simulink model "beta_estimator_acceleration"  (R2022a)
settings: Solver=VariableStepAuto  StartTime=0.0  StopTime=10.0  FixedStep=1e-3  RelTol=1e-6  AbsTol=1e-10
values from neighbouring files (symbols this model uses):
  Den_PDa = [1,(Ts/Ta-2)/(Ts/Ta+2)]    [test_beta_estimator_acceleration.m]    (also in test_beta_estimator_compare.m)
  Num_PDa = [(Kpa*(2+Ts/Ta)+2*Kda/Ta)/(2+Ts/Ta),(-2*Kpa+Ts*Kpa/Ta-2*Kda/Ta)/(2+Ts/Ta)]    [test_beta_estimator_acceleration.m]    (also in test_beta_estimator_compare.m)
  Ts = 0.001    [test_beta_estimator_acceleration.m]    (also in test_beta_estimator_compare.m; test_beta_estimator_velocity.m)
  x0_acc = [0,0,0,0.1]    [test_beta_estimator_acceleration.m]    (also in test_beta_estimator_compare.m)
undefined symbols (not defined in the file or in its folder): DiscIntNeverNeededParam
settings Model: Creator=bascetta  LastModifiedBy=bascetta
settings SolverCC: AlgebraicLoopSolver=TrustRegion
settings DataIOCC: SaveOutput=off  SignalLogging=off  DSMLogging=off  SaveTime=off  ReturnWorkspaceOutputs=off
settings OptimizationCC: DefaultParameterBehavior=Inlined  PassReuseOutputArgsAs=Individual arguments  MaxStackSize=64  EfficientTunableParamExpr=on
settings DebuggingCC: ParameterTunabilityLossMsg=error  UnconnectedInputMsg=warning  UnconnectedOutputMsg=warning  UnconnectedLineMsg=warning  SFMachineParentedDataDiag=warning  ArithmeticOperatorsInVariantConditions=warning
settings HardwareCC: ProdBitPerPointer=32  ProdBitPerSizeT=32  ProdBitPerPtrDiffT=32  ProdLargestAtomicFloat=None  ProdIntDivRoundTo=Undefined  ProdEndianess=Unspecified  ProdWordSize=32  ProdHWDeviceType=Generic->Unspecified (assume 32-bit Generic)
settings SFSimCC: SimUseLocalCustomCode=off  MATLABDynamicMemAlloc=off  CustomCodeUndefinedFunction=UseInterfaceOnly
settings RTWCC: SystemTargetFile=ert.tlc  TemplateMakefile=ert_default_tmf  GenerateReport=on  RTWUseLocalCustomCode=off  Toolchain=Catkin  IncludeHyperlinkInReport=on  LaunchReport=on  GenerateTraceInfo=on  GenerateTraceReport=on  GenerateTraceReportSl=on  GenerateTraceReportSf=on  GenerateTraceReportEml=on  DLArmComputeVersion=19.05
settings CodeAppCC: ForceParamTrailComments=on  IgnoreCustomStorageClasses=off  OperatorAnnotations=on  SimulinkDataObjDesc=on  SFDataObjDesc=on  MATLABFcnDesc=on  InsertBlockDesc=on  StateflowObjectComments=on  MATLABSourceComments=on
settings ERTTargetCC: ERTCustomFileTemplate=example_file_process.tlc

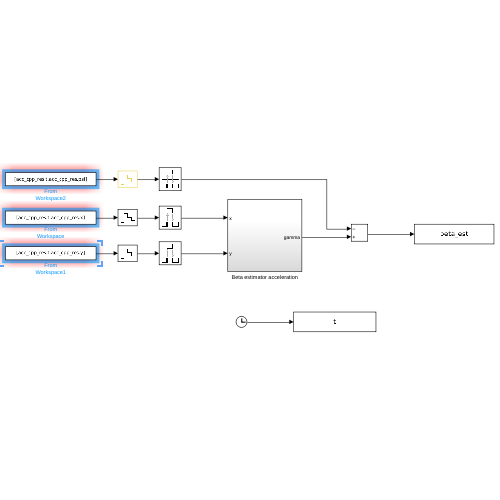
[thumbnail: Simulink's stored preview of the top-level diagram]
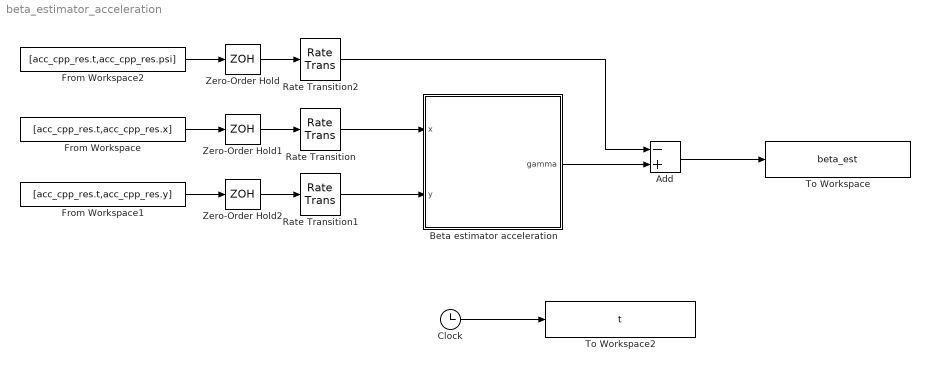
== system beta_estimator_acceleration ==
  Add : Sum  Inputs=-+
  Beta estimator acceleration : Subsystem  SystemSampleTime=Ts
  Clock : Clock
  From Workspace : FromWorkspace  VariableName=[acc_cpp_res.t,acc_cpp_res.x]  OutputAfterFinalValue=Holding final value
  From Workspace1 : FromWorkspace  VariableName=[acc_cpp_res.t,acc_cpp_res.y]  OutputAfterFinalValue=Holding final value
  From Workspace2 : FromWorkspace  VariableName=[acc_cpp_res.t,acc_cpp_res.psi]  OutputAfterFinalValue=Holding final value
  Rate Transition : RateTransition  OutPortSampleTime=Ts
  Rate Transition1 : RateTransition  OutPortSampleTime=Ts
  Rate Transition2 : RateTransition  OutPortSampleTime=Ts
  To Workspace : ToWorkspace  VariableName=beta_est  SampleTime=Ts
      settings: Save2DSignal=2-D array (concatenate along first dimension)
  To Workspace2 : ToWorkspace  VariableName=t  SampleTime=0.001
      settings: Save2DSignal=2-D array (concatenate along first dimension)
  Zero-Order Hold : ZeroOrderHold  SampleTime=0.01
  Zero-Order Hold1 : ZeroOrderHold  SampleTime=0.01
  Zero-Order Hold2 : ZeroOrderHold  SampleTime=0.01
  wires:
  Rate Transition/1 -> Beta estimator acceleration/1(x)
  Rate Transition1/1 -> Beta estimator acceleration/2(y)
  Beta estimator acceleration/1(gamma) -> Add/2
  Add/1 -> To Workspace/1
  Rate Transition2/1 -> Add/1
  Clock/1 -> To Workspace2/1
  From Workspace2/1 -> Zero-Order Hold/1
  Zero-Order Hold/1 -> Rate Transition2/1
  From Workspace/1 -> Zero-Order Hold1/1
  Zero-Order Hold1/1 -> Rate Transition/1
  From Workspace1/1 -> Zero-Order Hold2/1
  Zero-Order Hold2/1 -> Rate Transition1/1

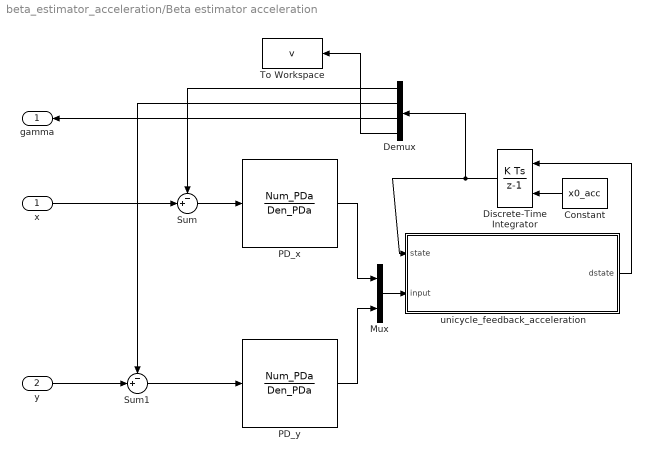
== system beta_estimator_acceleration/Beta estimator acceleration ==
  x : Inport
  y : Inport  Port=2
  Constant : Constant  Value=x0_acc
  Demux : Demux
  Discrete-Time Integrator : DiscreteIntegrator  InitialConditionSource=external  InitialCondition=[0 0 0 0.1]  SampleTime=Ts  ICPrevOutput=DiscIntNeverNeededParam  ICPrevScaledInput=DiscIntNeverNeededParam
  Mux : Mux  Inputs=2
  PD_x : DiscreteTransferFcn  Numerator=Num_PDa  Denominator=Den_PDa  SampleTime=Ts  a0EqualsOne=on
  PD_y : DiscreteTransferFcn  Numerator=Num_PDa  Denominator=Den_PDa  SampleTime=Ts  a0EqualsOne=on
  Sum : Sum  Inputs=-+|
  Sum1 : Sum  Inputs=-+|
  To Workspace : ToWorkspace  VariableName=v  SaveFormat=Timeseries  SampleTime=-1
  unicycle_feedback_acceleration : MATLAB Function  TreatAsAtomicUnit=on
  gamma : Outport  VectorParamsAs1DForOutWhenUnconnected=off
  wires:
  unicycle_feedback_acceleration/1(dstate) -> Discrete-Time Integrator/1
  Mux/1 -> unicycle_feedback_acceleration/2(input)
  Demux/1 -> Sum/1
  Sum/1 -> PD_x/1
  PD_x/1 -> Mux/1
  y/1 -> Sum1/2
  Demux/3 -> gamma/1
  Demux/2 -> Sum1/1
  Discrete-Time Integrator/1 -> unicycle_feedback_acceleration/1(state), Demux/1
  Demux/4 -> To Workspace/1
  x/1 -> Sum/2
  Sum1/1 -> PD_y/1
  PD_y/1 -> Mux/2
  Constant/1 -> Discrete-Time Integrator/2

== matlab function beta_estimator_acceleration/Beta estimator acceleration/unicycle_feedback_acceleration ==
  data: state input size=4; dstate output size=4; input input size=2
function dstate = unicycle_feedback_acceleration(state,input)

% State and input variables
x     = state(1); %[m]
y     = state(2); %[m]
gamma = state(3); % theta+beta [rad]
v     = state(4); %[m/s]

ax    = input(1); %[m/s^2]
ay    = input(2); %[m/s^2]

    % Model equations
    dstate = zeros(4,1);
    dstate(1) = v*cos(gamma); %dx/dt
    dstate(2) = v*sin(gamma); %dy/dt
    dstate(3) = (ay*cos(gamma)-ax*sin(gamma))/v; %d(gamma)/dt
    dstate(4) = ax*cos(gamma)+ay*sin(gamma); %dv/dt
end
